simulink model "V01_pendulum"  (R2018b)
settings: Solver=FixedStepAuto  StartTime=0.0  StopTime=10  FixedStep=0.001  RelTol=1e-3
model workspace (MAT data in the model file):
  J = 2
  L = 0.5
  M = 3
  g = 9.81
settings Model: Creator=Administrator  LastModifiedBy=Administrator

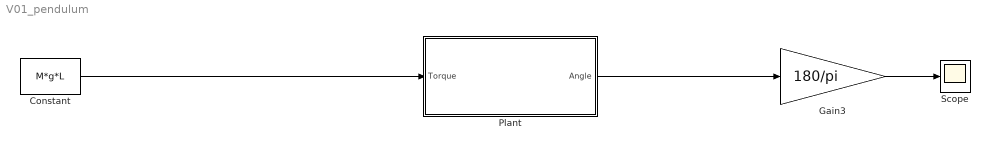
== system V01_pendulum ==
  Constant : Constant  Value=M*g*L
  Gain3 : Gain  Gain=180/pi
  Plant : Subsystem
  Scope : Scope
  wires:
  Gain3/1 -> Scope/1
  Constant/1 -> Plant/1(Torque)
  Plant/1(Angle) -> Gain3/1

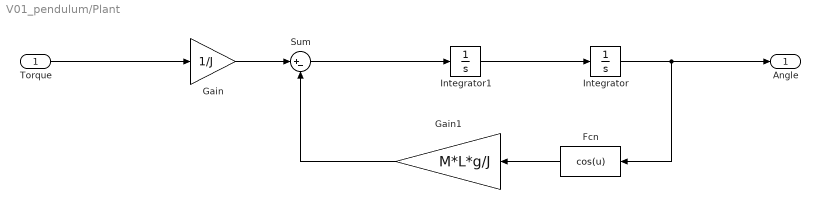
== system V01_pendulum/Plant ==
  Torque : Inport
  Fcn : Fcn  Expr=cos(u)
  Gain : Gain  Gain=1/J
  Gain1 : Gain  Gain=M*L*g/J
  Integrator : Integrator
  Integrator1 : Integrator
  Sum : Sum  Inputs=|+-
  Angle : Outport
  wires:
  Sum/1 -> Integrator1/1
  Gain1/1 -> Sum/2
  Fcn/1 -> Gain1/1
  Integrator1/1 -> Integrator/1
  Torque/1 -> Gain/1
  Gain/1 -> Sum/1
  Integrator/1 -> Angle/1, Fcn/1
